simulink library "HIL_GenSet"  (Simulink 7.8)
settings: Solver=ode45  StartTime=0.0  StopTime=10.0  RelTol=1e-3
values from neighbouring files (symbols this model uses):
  Ts = 80e-6    (= 8e-05)    [global_parameters.m]    (also in scopeBuffer.m)
undefined symbols (not defined in the file or in its folder): DiscIntNeverNeededParam, Ts_Power
libraries: simulink x77, powerlib x55, discretizing x28
(part 2 of 9)

== system HIL_GenSet/GenSet_3p5MW_RTLAB_07082015/Generator with  Primary Controllers ==
  note: Mirjana M: Parameters for this generators are preset parameters from SimPower System for 72.5kVAr
  wref : Inport
  Vtref : Inport  Port=2
  Enable : Inport  Port=3
  w_meas_Woodward : Inport  Port=4
  V_meas_Woodward : Inport  Port=5
  72.5 kva Diesel Engine Speed & Voltage Control fast : Subsystem
  Scope2 : Scope  NumInputPorts=2
      settings: YMin=0.949571~0.99979  YMax=1.04953~1  SaveName=ScopeData6
  Synchronous Machine pu Fundamental : powerlib/Machines/Synchronous Machine pu Fundamental  PresetModel=No  MechanicalLoad=Mechanical power Pm  ShowDetailedParameters=on  RotorType=Salient-pole  NominalParameters=[4.375+006 460 60]  Stator=[0.008979 0.05 2.35 1.72]  Field=[0.00206 0.511]  Dampers2=[0.0652, 0.5134, 0.0287, 0.2553, 7.765e-3, 0.9167 ]  Dampers1=[0.2826 3.738 0.02545 0.2392]  Mechanical=[0.3468 0.009238 2]  PolePairs=2  InitialConditions="[ 0  0  0  0  0  0  0  0  0 ]"  SetSaturation=off  Saturation=[0.6404,0.7127,0.8441,0.9214,0.9956,1.082,1.19,1.316,1.457;0.7,0.7698,0.8872,0.9466,0.9969,1.046,1.1,1.151,1.201]  Units=per unit fundamental parameters  LoadFlowParameters=[1,0,0,0,0]  TsPowergui=0  TsBlock=-1  IterativeModel=Forward Euler  BusType=PV  Pref=0  Qref=0  Qmin=-inf  Qmax=inf  PLF=0  QLF=0
  A : PMIOPort  Port=1  Side=Right
  B : PMIOPort  Port=2  Side=Right
  C : PMIOPort  Port=3  Side=Right
  m : Outport
  wires:
  Enable/1 -> 72.5 kva Diesel Engine Speed & Voltage Control fast/3(Generator Enable)
  Vtref/1 -> 72.5 kva Diesel Engine Speed & Voltage Control fast/2(Vtref)
  wref/1 -> 72.5 kva Diesel Engine Speed & Voltage Control fast/1(wref)
  72.5 kva Diesel Engine Speed & Voltage Control fast/3(Vt) -> Scope2/1  "vt"
  72.5 kva Diesel Engine Speed & Voltage Control fast/4(w) -> Scope2/2  "w"
  Synchronous Machine pu Fundamental/1 -> m/1, 72.5 kva Diesel Engine Speed & Voltage Control fast/4(m)
  72.5 kva Diesel Engine Speed & Voltage Control fast/2(Vf) -> Synchronous Machine pu Fundamental/2
  72.5 kva Diesel Engine Speed & Voltage Control fast/1(Pm) -> Synchronous Machine pu Fundamental/1
  w_meas_Woodward/1 -> 72.5 kva Diesel Engine Speed & Voltage Control fast/5(w_meas_Wood)
  V_meas_Woodward/1 -> 72.5 kva Diesel Engine Speed & Voltage Control fast/6(V_meas_Wood)
  connections:
  C/RConn1 -- Synchronous Machine pu Fundamental/RConn3
  B/RConn1 -- Synchronous Machine pu Fundamental/RConn2
  A/RConn1 -- Synchronous Machine pu Fundamental/RConn1

== system HIL_GenSet/GenSet_3p5MW_RTLAB_07082015/Interface between Woodward Controller and simated generator ==
  note: Note: This may need a different scaling because it is the reference signal.
      | Reference has to be between 0.95 and 1.05 pu in order to be in tolerance.
  Woodward for wref : Inport
  Woodward for Vref : Inport  Port=2
  Add2 : Sum
  Add3 : Sum
  Gain2 : Gain  Gain=0.01
  Gain3 : Gain  Gain=0.01
  Mux1 : Mux  Inputs=2
  Vref_set : Constant
  wref_set : Constant
  wref,Vref : Outport
  wires:
  Gain2/1 -> Add2/1  "bias"
  Add2/1 -> Mux1/1
  wref_set/1 -> Add2/2
  Gain3/1 -> Add3/1  "bias"
  Vref_set/1 -> Add3/2
  Add3/1 -> Mux1/2
  Woodward for wref/1 -> Gain2/1
  Mux1/1 -> wref,Vref/1  "hardware"
  Woodward for Vref/1 -> Gain3/1

== system HIL_GenSet/GenSet_3p5MW_RTLAB_07082015/Simulated Generator Controller 3.5 MW ==
  Pref : Inport
  Qref : Inport  Port=2
  mode : Inport  Port=3
  set_vtref : Inport  Port=4
  set_wref : Inport  Port=5
  gen_m : Inport  Port=6
  Bus Selector1 : BusSelector  OutputSignals="Output active power   Peo (pu),Output reactive power  Qeo (pu)"
  Multiport Switch : MultiPortSwitch  zeroidx=off
  Mux1 : Mux  Inputs=2
  Mux2 : Mux  Inputs=2
  Mux3 : Mux  Inputs=2
  PQ control : Subsystem
  PV control : Subsystem
  "wref, Vref" : Outport
  wires:
  Bus Selector1/1 -> PQ control/2(P (pu)), PV control/2(P (pu))  "<Output active power   Peo (pu)>"
  gen_m/1 -> Bus Selector1/1
  PQ control/1(w_ref (pu)) -> Mux1/1
  PQ control/2(V_ref (pu)) -> Mux1/2
  PV control/1(w_ref (pu)) -> Mux2/1
  set_vtref/1 -> Mux2/2, Mux3/2
  Mux1/1 -> Multiport Switch/2
  Mux2/1 -> Multiport Switch/3
  Mux3/1 -> Multiport Switch/4
  Pref/1 -> PQ control/1(P_ref (pu)), PV control/1(P_ref (pu))
  Bus Selector1/2 -> PQ control/4(Q (pu))  "<Output reactive power  Qeo (pu)>"
  set_wref/1 -> Mux3/1
  Qref/1 -> PQ control/3(Q_ref (pu))
  mode/1 -> Multiport Switch/1
  Multiport Switch/1 -> "wref, Vref"/1

== system HIL_GenSet/GenSet_3p5MW_nPID_Manual_RTLAB/Generator with  Primary Controllers ==
  wref : Inport
  Vtref : Inport  Port=2
  Enable : Inport  Port=3
  72.5 kva Diesel Engine Speed & Voltage Control fast : Subsystem
  Scope2 : Scope  NumInputPorts=2
      settings: YMin=0~0.93  YMax=1.05~1.12  SaveName=ScopeData6
  Synchronous Machine pu Fundamental : powerlib/Machines/Synchronous Machine pu Fundamental  PresetModel=No  MechanicalLoad=Mechanical power Pm  ShowDetailedParameters=on  RotorType=Salient-pole  NominalParameters=[4e+006 460 60]  Stator=[0.008979 0.05 2.35 1.72]  Field=[0.00206 0.511]  Dampers2=[0.0652, 0.5134, 0.0287, 0.2553, 7.765e-3, 0.9167 ]  Dampers1=[0.2826 3.738 0.02545 0.2392]  Mechanical=[0.3468 0.009238 2]  PolePairs=2  InitialConditions="[ 0  0  0  0  0  0  0  0  0 ]"  SetSaturation=off  Saturation=[0.6404,0.7127,0.8441,0.9214,0.9956,1.082,1.19,1.316,1.457;0.7,0.7698,0.8872,0.9466,0.9969,1.046,1.1,1.151,1.201]  Units=per unit fundamental parameters  LoadFlowParameters=[1,0,0,0,0]  TsPowergui=0  TsBlock=-1  IterativeModel=Forward Euler  BusType=PV  Pref=0  Qref=0  Qmin=-inf  Qmax=inf  PLF=0  QLF=0
  A : PMIOPort  Port=1  Side=Right
  B : PMIOPort  Port=2  Side=Right
  C : PMIOPort  Port=3  Side=Right
  m : Outport
  wires:
  Enable/1 -> 72.5 kva Diesel Engine Speed & Voltage Control fast/3(Generator Enable)
  Vtref/1 -> 72.5 kva Diesel Engine Speed & Voltage Control fast/2(Vtref)
  wref/1 -> 72.5 kva Diesel Engine Speed & Voltage Control fast/1(wref)
  72.5 kva Diesel Engine Speed & Voltage Control fast/3(Vt) -> Scope2/1  "vt"
  72.5 kva Diesel Engine Speed & Voltage Control fast/4(w) -> Scope2/2  "w"
  Synchronous Machine pu Fundamental/1 -> m/1, 72.5 kva Diesel Engine Speed & Voltage Control fast/4(m)
  72.5 kva Diesel Engine Speed & Voltage Control fast/2(Vf) -> Synchronous Machine pu Fundamental/2
  72.5 kva Diesel Engine Speed & Voltage Control fast/1(Pm) -> Synchronous Machine pu Fundamental/1
  connections:
  C/RConn1 -- Synchronous Machine pu Fundamental/RConn3
  B/RConn1 -- Synchronous Machine pu Fundamental/RConn2
  A/RConn1 -- Synchronous Machine pu Fundamental/RConn1

== system HIL_GenSet/GenSet_3p5MW_nPID_Manual_RTLAB/Simulated Generator Controller 3.5 MW ==
  Pref : Inport
  Qref : Inport  Port=2
  mode : Inport  Port=3
  set_vtref : Inport  Port=4
  set_wref : Inport  Port=5
  gen_m : Inport  Port=6
  Bus Selector1 : BusSelector  OutputSignals="Output active power   Peo (pu),Output reactive power  Qeo (pu)"
  Multiport Switch : MultiPortSwitch  zeroidx=off
  Mux1 : Mux  Inputs=2
  Mux2 : Mux  Inputs=2
  Mux3 : Mux  Inputs=2
  PQ control : Subsystem
  PV control : Subsystem
  "wref, Vref" : Outport
  wires:
  Bus Selector1/1 -> PQ control/2(P (pu)), PV control/2(P (pu))  "<Output active power   Peo (pu)>"
  gen_m/1 -> Bus Selector1/1
  PQ control/1(w_ref (pu)) -> Mux1/1
  PQ control/2(V_ref (pu)) -> Mux1/2
  PV control/1(w_ref (pu)) -> Mux2/1
  set_vtref/1 -> Mux2/2, Mux3/2
  Mux1/1 -> Multiport Switch/2
  Mux2/1 -> Multiport Switch/3
  Mux3/1 -> Multiport Switch/4
  Pref/1 -> PQ control/1(P_ref (pu)), PV control/1(P_ref (pu))
  Bus Selector1/2 -> PQ control/4(Q (pu))  "<Output reactive power  Qeo (pu)>"
  set_wref/1 -> Mux3/1
  Qref/1 -> PQ control/3(Q_ref (pu))
  mode/1 -> Multiport Switch/1
  Multiport Switch/1 -> "wref, Vref"/1

== system HIL_GenSet/GenSet_3p5MW_new_PID_RTLAB/60kW Generator with  Primary Controllers ==
  note: Mirjana M: Parameters for this generators are preset parameters from SimPower System for 72.5kVAr
  wref : Inport
  Vtref : Inport  Port=2
  Enable : Inport  Port=3
  w_meas_Woodward : Inport  Port=4
  V_meas_Woodward : Inport  Port=5
  72.5 kva Diesel Engine Speed & Voltage Control fast : Subsystem
  Scope2 : Scope  NumInputPorts=2
      settings: YMin=0.949571~0.99979  YMax=1.04953~1  SaveName=ScopeData6
  Synchronous Machine pu Fundamental : powerlib/Machines/Synchronous Machine pu Fundamental  PresetModel=No  MechanicalLoad=Mechanical power Pm  ShowDetailedParameters=on  RotorType=Salient-pole  NominalParameters=[4.375+006 460 60]  Stator=[0.008979 0.05 2.35 1.72]  Field=[0.00206 0.511]  Dampers2=[0.0652, 0.5134, 0.0287, 0.2553, 7.765e-3, 0.9167 ]  Dampers1=[0.2826 3.738 0.02545 0.2392]  Mechanical=[0.3468 0.009238 2]  PolePairs=2  InitialConditions="[ 0  0  0  0  0  0  0  0  0 ]"  SetSaturation=off  Saturation=[0.6404,0.7127,0.8441,0.9214,0.9956,1.082,1.19,1.316,1.457;0.7,0.7698,0.8872,0.9466,0.9969,1.046,1.1,1.151,1.201]  Units=per unit fundamental parameters  LoadFlowParameters=[1,0,0,0,0]  TsPowergui=0  TsBlock=-1  IterativeModel=Forward Euler  BusType=PV  Pref=0  Qref=0  Qmin=-inf  Qmax=inf  PLF=0  QLF=0
  A : PMIOPort  Port=1  Side=Right
  B : PMIOPort  Port=2  Side=Right
  C : PMIOPort  Port=3  Side=Right
  m : Outport
  wires:
  Enable/1 -> 72.5 kva Diesel Engine Speed & Voltage Control fast/3(Generator Enable)
  Vtref/1 -> 72.5 kva Diesel Engine Speed & Voltage Control fast/2(Vtref)
  wref/1 -> 72.5 kva Diesel Engine Speed & Voltage Control fast/1(wref)
  72.5 kva Diesel Engine Speed & Voltage Control fast/3(Vt) -> Scope2/1
  72.5 kva Diesel Engine Speed & Voltage Control fast/4(w) -> Scope2/2
  Synchronous Machine pu Fundamental/1 -> m/1, 72.5 kva Diesel Engine Speed & Voltage Control fast/4(m)
  72.5 kva Diesel Engine Speed & Voltage Control fast/2(Vf) -> Synchronous Machine pu Fundamental/2
  72.5 kva Diesel Engine Speed & Voltage Control fast/1(Pm) -> Synchronous Machine pu Fundamental/1
  w_meas_Woodward/1 -> 72.5 kva Diesel Engine Speed & Voltage Control fast/5(w_meas_Wood)
  V_meas_Woodward/1 -> 72.5 kva Diesel Engine Speed & Voltage Control fast/6(V_meas_Wood)
  connections:
  C/RConn1 -- Synchronous Machine pu Fundamental/RConn3
  B/RConn1 -- Synchronous Machine pu Fundamental/RConn2
  A/RConn1 -- Synchronous Machine pu Fundamental/RConn1

== system HIL_GenSet/GenSet_3p5MW_new_PID_RTLAB/Interface between Woodward Controller and simated generator ==
  note: Note: This may need a different scaling because it is the reference signal.
      | Reference has to be between 0.95 and 1.05 pu in order to be in tolerance.
  Woodward for wref : Inport
  Woodward for Vref : Inport  Port=2
  Add2 : Sum
  Add3 : Sum
  Gain2 : Gain  Gain=0.005
  Gain3 : Gain  Gain=0.005
  Mux1 : Mux  Inputs=2
  Vref_set : Constant
  wref_set : Constant
  wref,Vref : Outport
  wires:
  Gain2/1 -> Add2/1  "bias"
  Add2/1 -> Mux1/1
  wref_set/1 -> Add2/2
  Gain3/1 -> Add3/1  "bias"
  Vref_set/1 -> Add3/2
  Add3/1 -> Mux1/2
  Woodward for wref/1 -> Gain2/1
  Mux1/1 -> wref,Vref/1  "hardware"
  Woodward for Vref/1 -> Gain3/1

== system HIL_GenSet/GenSet_3p5MW_new_PID_RTLAB/Simulated Generator Controller ==
  Bus Selector1 : BusSelector  OutputSignals="Output active power   Peo (pu),Output reactive power  Qeo (pu)"
  Multiport Switch : MultiPortSwitch  zeroidx=off
  Mux1 : Mux  Inputs=2
  Mux2 : Mux  Inputs=2
  Mux3 : Mux  Inputs=2
  PQ control : Subsystem
  PV control : Subsystem
  Pref : Constant  Value=set_Pref
  Qref : Constant  Value=set_Qref
  mode (1-3) : Constant  Value=mode
  set_vtref : Constant  Value=set_vref
  set_wref : Constant  Value=set_wref
  "wref, Vref" : Outport
  wires:
  Bus Selector1/1 -> PQ control/2(P (pu)), PV control/2(P (pu))  "<Output active power   Peo (pu)>"
  [gen_m] -> Bus Selector1/1
  PQ control/1(w_ref (pu)) -> Mux1/1
  PQ control/2(V_ref (pu)) -> Mux1/2
  PV control/1(w_ref (pu)) -> Mux2/1
  set_vtref/1 -> Mux2/2, Mux3/2
  Mux1/1 -> Multiport Switch/2
  Mux2/1 -> Multiport Switch/3
  Mux3/1 -> Multiport Switch/4
  Pref/1 -> PQ control/1(P_ref (pu)), PV control/1(P_ref (pu))
  Bus Selector1/2 -> PQ control/4(Q (pu))  "<Output reactive power  Qeo (pu)>"
  set_wref/1 -> Mux3/1
  Qref/1 -> PQ control/3(Q_ref (pu))
  mode (1-3)/1 -> Multiport Switch/1
  Multiport Switch/1 -> "wref, Vref"/1

== system HIL_GenSet/GenSet_4MW_14kV/Generator with  Primary Controllers ==
  wref : Inport
  Vtref : Inport  Port=2
  Enable : Inport  Port=3
  72.5 kva Diesel Engine Speed & Voltage Control fast : Subsystem
  Synchronous Machine pu Fundamental : powerlib/Machines/Synchronous Machine pu Fundamental  PresetModel=No  MechanicalLoad=Mechanical power Pm  ShowDetailedParameters=on  RotorType=Salient-pole  NominalParameters=[4e+006 13800 60]  Stator=[0.008979 0.05 2.35 1.72]  Field=[0.00206 0.511]  Dampers2=[0.0652, 0.5134, 0.0287, 0.2553, 7.765e-3, 0.9167 ]  Dampers1=[0.2826 3.738 0.02545 0.2392]  Mechanical=[0.3468 0.009238 2]  PolePairs=2  InitialConditions="[ 0  0  0  0  0  0  0  0  0 ]"  SetSaturation=off  Saturation=[0.6404,0.7127,0.8441,0.9214,0.9956,1.082,1.19,1.316,1.457;0.7,0.7698,0.8872,0.9466,0.9969,1.046,1.1,1.151,1.201]  Units=per unit fundamental parameters  LoadFlowParameters=[1,0,0,0,0]  TsPowergui=0  TsBlock=-1  IterativeModel=Forward Euler  BusType=PV  Pref=0  Qref=0  Qmin=-inf  Qmax=inf  PLF=0  QLF=0
  Terminator : Terminator
  Terminator1 : Terminator
  A : PMIOPort  Port=1  Side=Right
  B : PMIOPort  Port=2  Side=Right
  C : PMIOPort  Port=3  Side=Right
  m : Outport
  wires:
  Enable/1 -> 72.5 kva Diesel Engine Speed & Voltage Control fast/3(Generator Enable)
  Vtref/1 -> 72.5 kva Diesel Engine Speed & Voltage Control fast/2(Vtref)
  wref/1 -> 72.5 kva Diesel Engine Speed & Voltage Control fast/1(wref)
  Synchronous Machine pu Fundamental/1 -> m/1, 72.5 kva Diesel Engine Speed & Voltage Control fast/4(m)
  72.5 kva Diesel Engine Speed & Voltage Control fast/2(Vf) -> Synchronous Machine pu Fundamental/2
  72.5 kva Diesel Engine Speed & Voltage Control fast/1(Pm) -> Synchronous Machine pu Fundamental/1
  72.5 kva Diesel Engine Speed & Voltage Control fast/3(Vt) -> Terminator/1  "vt"
  72.5 kva Diesel Engine Speed & Voltage Control fast/4(w) -> Terminator1/1  "w"
  connections:
  C/RConn1 -- Synchronous Machine pu Fundamental/RConn3
  B/RConn1 -- Synchronous Machine pu Fundamental/RConn2
  A/RConn1 -- Synchronous Machine pu Fundamental/RConn1

== system HIL_GenSet/GenSet_4MW_14kV/NumOscillation ==
  Ground2 : powerlib/Elements/Ground  LConnTagsString=a
  "RLC " : powerlib/Elements/Parallel RLC Branch  LConnTagsString=a  RConnTagsString=__new0  BranchType=R  Resistance=10e6  Inductance=inf  SetiL0=off  InitialCurrent=0  Capacitance=10e-6  Setx0=off  InitialVoltage=0  Measurements=None
  RLC1 : powerlib/Elements/Parallel RLC Branch  LConnTagsString=a  RConnTagsString=__new0  BranchType=R  Resistance=10e6  Inductance=inf  SetiL0=off  InitialCurrent=0  Capacitance=10e-6  Setx0=off  InitialVoltage=0  Measurements=None
  RLC2 : powerlib/Elements/Parallel RLC Branch  LConnTagsString=a  RConnTagsString=__new0  BranchType=R  Resistance=10e6  Inductance=inf  SetiL0=off  InitialCurrent=0  Capacitance=10e-6  Setx0=off  InitialVoltage=0  Measurements=None
  RLC3 : powerlib/Elements/Parallel RLC Branch  LConnTagsString=a  RConnTagsString=__new0  BranchType=R  Resistance=10e-3  Inductance=inf  SetiL0=off  InitialCurrent=0  Capacitance=0  Setx0=off  InitialVoltage=0  Measurements=None
  RLC4 : powerlib/Elements/Parallel RLC Branch  LConnTagsString=a  RConnTagsString=__new0  BranchType=R  Resistance=10e-3  Inductance=inf  SetiL0=off  InitialCurrent=0  Capacitance=0  Setx0=off  InitialVoltage=0  Measurements=None
  RLC5 : powerlib/Elements/Parallel RLC Branch  LConnTagsString=a  RConnTagsString=__new0  BranchType=R  Resistance=10e-3  Inductance=inf  SetiL0=off  InitialCurrent=0  Capacitance=0  Setx0=off  InitialVoltage=0  Measurements=None
  A : PMIOPort  Port=1  Side=Left
  B : PMIOPort  Port=2  Side=Left
  C : PMIOPort  Port=3  Side=Left
  connections:
  C/RConn1 -- RLC5/LConn1
  B/RConn1 -- RLC4/LConn1
  A/RConn1 -- RLC3/LConn1
  RLC3/RConn1 -- RLC2/LConn1
  RLC1/LConn1 -- RLC4/RConn1
  "RLC "/LConn1 -- RLC5/RConn1
  RLC2/RConn1 -- Ground2/LConn1 -- RLC1/RConn1 -- "RLC "/RConn1

== system HIL_GenSet/GenSet_4MW_14kV/Simulated Generator Controller 3.5 MW ==
  Pref : Inport
  Qref : Inport  Port=2
  mode : Inport  Port=3
  set_vtref : Inport  Port=4
  set_wref : Inport  Port=5
  gen_m : Inport  Port=6
  Bus Selector1 : BusSelector  OutputSignals="Output active power   Peo (pu),Output reactive power  Qeo (pu)"
  Multiport Switch : MultiPortSwitch  zeroidx=off
  Mux1 : Mux  Inputs=2
  Mux2 : Mux  Inputs=2
  Mux3 : Mux  Inputs=2
  PQ control : Subsystem
  PV control : Subsystem
  "wref, Vref" : Outport
  wires:
  Bus Selector1/1 -> PQ control/2(P (pu)), PV control/2(P (pu))  "<Output active power   Peo (pu)>"
  gen_m/1 -> Bus Selector1/1
  PQ control/1(w_ref (pu)) -> Mux1/1
  PQ control/2(V_ref (pu)) -> Mux1/2
  PV control/1(w_ref (pu)) -> Mux2/1
  set_vtref/1 -> Mux2/2, Mux3/2
  Mux1/1 -> Multiport Switch/2
  Mux2/1 -> Multiport Switch/3
  Mux3/1 -> Multiport Switch/4
  Pref/1 -> PQ control/1(P_ref (pu)), PV control/1(P_ref (pu))
  Bus Selector1/2 -> PQ control/4(Q (pu))  "<Output reactive power  Qeo (pu)>"
  set_wref/1 -> Mux3/1
  Qref/1 -> PQ control/3(Q_ref (pu))
  mode/1 -> Multiport Switch/1
  Multiport Switch/1 -> "wref, Vref"/1

== system HIL_GenSet/GenSet_4MW_14kV_07232015/Generator with  Primary Controllers ==
  wref : Inport
  Vtref : Inport  Port=2
  Enable : Inport  Port=3
  Diesel Engine Speed & Voltage Control fast : Subsystem
  Synchronous Machine pu Fundamental : powerlib/Machines/Synchronous Machine pu Fundamental  PresetModel=No  MechanicalLoad=Mechanical power Pm  ShowDetailedParameters=on  RotorType=Salient-pole  NominalParameters=[4e+006 13800 60]  Stator=[0.008979 0.05 2.35 1.72]  Field=[0.00206 0.511]  Dampers2=[0.0652, 0.5134, 0.0287, 0.2553, 7.765e-3, 0.9167 ]  Dampers1=[0.2826 3.738 0.02545 0.2392]  Mechanical=[0.3468 0.009238 2]  PolePairs=2  InitialConditions="[ 0  0  0  0  0  0  0  0  0 ]"  SetSaturation=off  Saturation=[0.6404,0.7127,0.8441,0.9214,0.9956,1.082,1.19,1.316,1.457;0.7,0.7698,0.8872,0.9466,0.9969,1.046,1.1,1.151,1.201]  Units=per unit fundamental parameters  LoadFlowParameters=[1,0,0,0,0]  TsPowergui=0  TsBlock=-1  IterativeModel=Forward Euler  BusType=PV  Pref=0  Qref=0  Qmin=-inf  Qmax=inf  PLF=0  QLF=0
  Terminator : Terminator
  Terminator1 : Terminator
  A : PMIOPort  Port=1  Side=Right
  B : PMIOPort  Port=2  Side=Right
  C : PMIOPort  Port=3  Side=Right
  m : Outport
  wires:
  Enable/1 -> Diesel Engine Speed & Voltage Control fast/3(Generator Enable)
  Vtref/1 -> Diesel Engine Speed & Voltage Control fast/2(Vtref)
  wref/1 -> Diesel Engine Speed & Voltage Control fast/1(wref)
  Synchronous Machine pu Fundamental/1 -> m/1, Diesel Engine Speed & Voltage Control fast/4(m)
  Diesel Engine Speed & Voltage Control fast/2(Vf) -> Synchronous Machine pu Fundamental/2
  Diesel Engine Speed & Voltage Control fast/1(Pm) -> Synchronous Machine pu Fundamental/1
  Diesel Engine Speed & Voltage Control fast/3(Vt) -> Terminator/1  "vt"
  Diesel Engine Speed & Voltage Control fast/4(w) -> Terminator1/1  "w"
  connections:
  C/RConn1 -- Synchronous Machine pu Fundamental/RConn3
  B/RConn1 -- Synchronous Machine pu Fundamental/RConn2
  A/RConn1 -- Synchronous Machine pu Fundamental/RConn1

== system HIL_GenSet/GenSet_4MW_14kV_07232015/NumOscillation ==
  Ground2 : powerlib/Elements/Ground  LConnTagsString=a
  "RLC " : powerlib/Elements/Parallel RLC Branch  LConnTagsString=a  RConnTagsString=__new0  BranchType=R  Resistance=10e6  Inductance=inf  SetiL0=off  InitialCurrent=0  Capacitance=10e-6  Setx0=off  InitialVoltage=0  Measurements=None
  RLC1 : powerlib/Elements/Parallel RLC Branch  LConnTagsString=a  RConnTagsString=__new0  BranchType=R  Resistance=10e6  Inductance=inf  SetiL0=off  InitialCurrent=0  Capacitance=10e-6  Setx0=off  InitialVoltage=0  Measurements=None
  RLC2 : powerlib/Elements/Parallel RLC Branch  LConnTagsString=a  RConnTagsString=__new0  BranchType=R  Resistance=10e6  Inductance=inf  SetiL0=off  InitialCurrent=0  Capacitance=10e-6  Setx0=off  InitialVoltage=0  Measurements=None
  RLC3 : powerlib/Elements/Parallel RLC Branch  LConnTagsString=a  RConnTagsString=__new0  BranchType=R  Resistance=10e-3  Inductance=inf  SetiL0=off  InitialCurrent=0  Capacitance=0  Setx0=off  InitialVoltage=0  Measurements=None
  RLC4 : powerlib/Elements/Parallel RLC Branch  LConnTagsString=a  RConnTagsString=__new0  BranchType=R  Resistance=10e-3  Inductance=inf  SetiL0=off  InitialCurrent=0  Capacitance=0  Setx0=off  InitialVoltage=0  Measurements=None
  RLC5 : powerlib/Elements/Parallel RLC Branch  LConnTagsString=a  RConnTagsString=__new0  BranchType=R  Resistance=10e-3  Inductance=inf  SetiL0=off  InitialCurrent=0  Capacitance=0  Setx0=off  InitialVoltage=0  Measurements=None
  A : PMIOPort  Port=1  Side=Left
  B : PMIOPort  Port=2  Side=Left
  C : PMIOPort  Port=3  Side=Left
  connections:
  C/RConn1 -- RLC5/LConn1
  B/RConn1 -- RLC4/LConn1
  A/RConn1 -- RLC3/LConn1
  RLC3/RConn1 -- RLC2/LConn1
  RLC1/LConn1 -- RLC4/RConn1
  "RLC "/LConn1 -- RLC5/RConn1
  RLC2/RConn1 -- Ground2/LConn1 -- RLC1/RConn1 -- "RLC "/RConn1

== system HIL_GenSet/GenSet_4MW_14kV_07232015/Simulated Generator Controller 3.5 MW ==
  Pref : Inport
  Qref : Inport  Port=2
  mode : Inport  Port=3
  set_vtref : Inport  Port=4
  set_wref : Inport  Port=5
  gen_m : Inport  Port=6
  Bus Selector1 : BusSelector  OutputSignals="Output active power   Peo (pu),Output reactive power  Qeo (pu)"
  Multiport Switch : MultiPortSwitch  zeroidx=off
  Mux1 : Mux  Inputs=2
  Mux2 : Mux  Inputs=2
  Mux3 : Mux  Inputs=2
  PQ control : Subsystem
  PV control : Subsystem
  "wref, Vref" : Outport
  wires:
  Bus Selector1/1 -> PQ control/2(P (pu)), PV control/2(P (pu))  "<Output active power   Peo (pu)>"
  gen_m/1 -> Bus Selector1/1
  PQ control/1(w_ref (pu)) -> Mux1/1
  PQ control/2(V_ref (pu)) -> Mux1/2
  PV control/1(w_ref (pu)) -> Mux2/1
  set_vtref/1 -> Mux2/2, Mux3/2
  Mux1/1 -> Multiport Switch/2
  Mux2/1 -> Multiport Switch/3
  Mux3/1 -> Multiport Switch/4
  Pref/1 -> PQ control/1(P_ref (pu)), PV control/1(P_ref (pu))
  Bus Selector1/2 -> PQ control/4(Q (pu))  "<Output reactive power  Qeo (pu)>"
  set_wref/1 -> Mux3/1
  Qref/1 -> PQ control/3(Q_ref (pu))
  mode/1 -> Multiport Switch/1
  Multiport Switch/1 -> "wref, Vref"/1

== system HIL_GenSet/GenSet_4MW_14kV_07232015/StabilityL ==
  Constant Load : powerlib/Elements/Three-Phase Parallel RLC Load  LConnTagsString=A|B|C  Configuration=Y (grounded)  NominalVoltage=v  NominalFrequency=60  ActivePower=kVA*1E3*pf  InductivePower=kVA*1E3*sqrt(1-pf^2)  CapacitivePower=0  Measurements=None  LoadType=constant Z
  A : PMIOPort  Port=1  Side=Left
  B : PMIOPort  Port=2  Side=Left
  C : PMIOPort  Port=3  Side=Left
  connections:
  A/RConn1 -- Constant Load/LConn1
  B/RConn1 -- Constant Load/LConn2
  C/RConn1 -- Constant Load/LConn3

== system HIL_GenSet/GenSet_4MW_14kV_09022015/Generator with  Primary Controllers ==
  wref : Inport
  Vtref : Inport  Port=2
  Enable : Inport  Port=3
  Diesel Engine Speed & Voltage Control fast : Subsystem
  Synchronous Machine pu Fundamental : powerlib/Machines/Synchronous Machine pu Fundamental  PresetModel=No  MechanicalLoad=Mechanical power Pm  ShowDetailedParameters=on  RotorType=Salient-pole  NominalParameters=[4e+006 13800 60]  Stator=[0.008979 0.05 2.35 1.72]  Field=[0.00206 0.511]  Dampers2=[0.0652, 0.5134, 0.0287, 0.2553, 7.765e-3, 0.9167 ]  Dampers1=[0.2826 3.738 0.02545 0.2392]  Mechanical=[0.3468 0.009238 2]  PolePairs=2  InitialConditions="[ 0  0  0  0  0  0  0  0  0 ]"  SetSaturation=off  Saturation=[0.6404,0.7127,0.8441,0.9214,0.9956,1.082,1.19,1.316,1.457;0.7,0.7698,0.8872,0.9466,0.9969,1.046,1.1,1.151,1.201]  Units=per unit fundamental parameters  LoadFlowParameters=[1,0,0,0,0]  TsPowergui=0  TsBlock=-1  IterativeModel=Forward Euler  BusType=PV  Pref=0  Qref=0  Qmin=-inf  Qmax=inf  PLF=0  QLF=0
  Terminator : Terminator
  Terminator1 : Terminator
  A : PMIOPort  Port=1  Side=Right
  B : PMIOPort  Port=2  Side=Right
  C : PMIOPort  Port=3  Side=Right
  m : Outport
  wires:
  Enable/1 -> Diesel Engine Speed & Voltage Control fast/3(Generator Enable)
  Vtref/1 -> Diesel Engine Speed & Voltage Control fast/2(Vtref)
  wref/1 -> Diesel Engine Speed & Voltage Control fast/1(wref)
  Synchronous Machine pu Fundamental/1 -> m/1, Diesel Engine Speed & Voltage Control fast/4(m)
  Diesel Engine Speed & Voltage Control fast/2(Vf) -> Synchronous Machine pu Fundamental/2
  Diesel Engine Speed & Voltage Control fast/1(Pm) -> Synchronous Machine pu Fundamental/1
  Diesel Engine Speed & Voltage Control fast/3(Vt) -> Terminator/1  "vt"
  Diesel Engine Speed & Voltage Control fast/4(w) -> Terminator1/1  "w"
  connections:
  C/RConn1 -- Synchronous Machine pu Fundamental/RConn3
  B/RConn1 -- Synchronous Machine pu Fundamental/RConn2
  A/RConn1 -- Synchronous Machine pu Fundamental/RConn1

== system HIL_GenSet/GenSet_4MW_14kV_09022015/NumOscillation ==
  Ground2 : powerlib/Elements/Ground  LConnTagsString=a
  "RLC " : powerlib/Elements/Parallel RLC Branch  LConnTagsString=a  RConnTagsString=__new0  BranchType=R  Resistance=10e6  Inductance=inf  SetiL0=off  InitialCurrent=0  Capacitance=10e-6  Setx0=off  InitialVoltage=0  Measurements=None
  RLC1 : powerlib/Elements/Parallel RLC Branch  LConnTagsString=a  RConnTagsString=__new0  BranchType=R  Resistance=10e6  Inductance=inf  SetiL0=off  InitialCurrent=0  Capacitance=10e-6  Setx0=off  InitialVoltage=0  Measurements=None
  RLC2 : powerlib/Elements/Parallel RLC Branch  LConnTagsString=a  RConnTagsString=__new0  BranchType=R  Resistance=10e6  Inductance=inf  SetiL0=off  InitialCurrent=0  Capacitance=10e-6  Setx0=off  InitialVoltage=0  Measurements=None
  RLC3 : powerlib/Elements/Parallel RLC Branch  LConnTagsString=a  RConnTagsString=__new0  BranchType=R  Resistance=10e-3  Inductance=inf  SetiL0=off  InitialCurrent=0  Capacitance=0  Setx0=off  InitialVoltage=0  Measurements=None
  RLC4 : powerlib/Elements/Parallel RLC Branch  LConnTagsString=a  RConnTagsString=__new0  BranchType=R  Resistance=10e-3  Inductance=inf  SetiL0=off  InitialCurrent=0  Capacitance=0  Setx0=off  InitialVoltage=0  Measurements=None
  RLC5 : powerlib/Elements/Parallel RLC Branch  LConnTagsString=a  RConnTagsString=__new0  BranchType=R  Resistance=10e-3  Inductance=inf  SetiL0=off  InitialCurrent=0  Capacitance=0  Setx0=off  InitialVoltage=0  Measurements=None
  A : PMIOPort  Port=1  Side=Left
  B : PMIOPort  Port=2  Side=Left
  C : PMIOPort  Port=3  Side=Left
  connections:
  C/RConn1 -- RLC5/LConn1
  B/RConn1 -- RLC4/LConn1
  A/RConn1 -- RLC3/LConn1
  RLC3/RConn1 -- RLC2/LConn1
  RLC1/LConn1 -- RLC4/RConn1
  "RLC "/LConn1 -- RLC5/RConn1
  RLC2/RConn1 -- Ground2/LConn1 -- RLC1/RConn1 -- "RLC "/RConn1

== system HIL_GenSet/GenSet_4MW_14kV_09022015/Simulated Generator Controller 3.5 MW ==
  Pref : Inport
  Qref : Inport  Port=2
  mode : Inport  Port=3
  set_vtref : Inport  Port=4
  set_wref : Inport  Port=5
  gen_m : Inport  Port=6
  Bus Selector1 : BusSelector  OutputSignals="Output active power   Peo (pu),Output reactive power  Qeo (pu)"
  Multiport Switch : MultiPortSwitch  zeroidx=off
  Mux1 : Mux  Inputs=2
  Mux2 : Mux  Inputs=2
  Mux3 : Mux  Inputs=2
  PQ control : Subsystem
  PV control : Subsystem
  "wref, Vref" : Outport
  wires:
  Bus Selector1/1 -> PQ control/2(P (pu)), PV control/2(P (pu))  "<Output active power   Peo (pu)>"
  gen_m/1 -> Bus Selector1/1
  PQ control/1(w_ref (pu)) -> Mux1/1
  PQ control/2(V_ref (pu)) -> Mux1/2
  PV control/1(w_ref (pu)) -> Mux2/1
  set_vtref/1 -> Mux2/2, Mux3/2
  Mux1/1 -> Multiport Switch/2
  Mux2/1 -> Multiport Switch/3
  Mux3/1 -> Multiport Switch/4
  Pref/1 -> PQ control/1(P_ref (pu)), PV control/1(P_ref (pu))
  Bus Selector1/2 -> PQ control/4(Q (pu))  "<Output reactive power  Qeo (pu)>"
  set_wref/1 -> Mux3/1
  Qref/1 -> PQ control/3(Q_ref (pu))
  mode/1 -> Multiport Switch/1
  Multiport Switch/1 -> "wref, Vref"/1

== system HIL_GenSet/GenSet_4MW_14kV_09022015/StabilityL ==
  Constant Load : powerlib/Elements/Three-Phase Parallel RLC Load  LConnTagsString=A|B|C  Configuration=Y (grounded)  NominalVoltage=v  NominalFrequency=60  ActivePower=kVA*1E3*pf  InductivePower=kVA*1E3*sqrt(1-pf^2)  CapacitivePower=0  Measurements=None  LoadType=constant Z
  A : PMIOPort  Port=1  Side=Left
  B : PMIOPort  Port=2  Side=Left
  C : PMIOPort  Port=3  Side=Left
  connections:
  A/RConn1 -- Constant Load/LConn1
  B/RConn1 -- Constant Load/LConn2
  C/RConn1 -- Constant Load/LConn3

== system HIL_GenSet/GenSet_900kW_07232015/900kW Generator with  Primary Controllers ==
  note: Mirjana M: Parameters for this generators are preset parameters from SimPower System for 72.5kVAr
  wref : Inport
  Vtref : Inport  Port=2
  Enable : Inport  Port=3
  w_meas_Woodward : Inport  Port=4
  V_meas_Woodward : Inport  Port=5
  Diesel Engine Speed & Voltage Control fast : Subsystem
  Synchronous Machine pu Fundamental : powerlib/Machines/Synchronous Machine pu Fundamental  PresetModel=22: 60Hz 460V 1075kVA 1800RPM  MechanicalLoad=Mechanical power Pm  ShowDetailedParameters=on  RotorType=Salient-pole  NominalParameters=[1.075e+006 460 60]  Stator=[0.01524 0.08 2.81 1.64]  Field=[0.004319 0.531]  Dampers2=[0.0652, 0.5134, 0.0287, 0.2553, 7.765e-3, 0.9167 ]  Dampers1=[0.2343 2.655 0.03365 0.2408]  Mechanical=[0.3222 0.01322 2]  PolePairs=2  InitialConditions="[ 0  0  0  0  0  0  0  0  0 ]"  SetSaturation=off  Saturation=[0.6404,0.7127,0.8441,0.9214,0.9956,1.082,1.19,1.316,1.457;0.7,0.7698,0.8872,0.9466,0.9969,1.046,1.1,1.151,1.201]  Units=per unit fundamental parameters  LoadFlowParameters=[1,0,0,0,0]  TsPowergui=0  TsBlock=-1  IterativeModel=Forward Euler  BusType=PV  Pref=0  Qref=0  Qmin=-inf  Qmax=inf  PLF=0  QLF=0
  Terminator : Terminator
  Terminator1 : Terminator
  A : PMIOPort  Port=1  Side=Right
  B : PMIOPort  Port=2  Side=Right
  C : PMIOPort  Port=3  Side=Right
  m : Outport
  wires:
  Diesel Engine Speed & Voltage Control fast/4(w) -> Terminator1/1  "w"
  Diesel Engine Speed & Voltage Control fast/3(Vt) -> Terminator/1  "vt"
  Vtref/1 -> Diesel Engine Speed & Voltage Control fast/2(Vtref)
  wref/1 -> Diesel Engine Speed & Voltage Control fast/1(wref)
  Diesel Engine Speed & Voltage Control fast/2(Vf) -> Synchronous Machine pu Fundamental/2  "vf"
  Diesel Engine Speed & Voltage Control fast/1(Pm) -> Synchronous Machine pu Fundamental/1  "pm"
  Enable/1 -> Diesel Engine Speed & Voltage Control fast/3(Generator Enable)
  Synchronous Machine pu Fundamental/1 -> m/1, Diesel Engine Speed & Voltage Control fast/4(m)
  w_meas_Woodward/1 -> Diesel Engine Speed & Voltage Control fast/5(w_meas_Wood)
  V_meas_Woodward/1 -> Diesel Engine Speed & Voltage Control fast/6(V_meas_Wood)
  connections:
  C/RConn1 -- Synchronous Machine pu Fundamental/RConn3
  B/RConn1 -- Synchronous Machine pu Fundamental/RConn2
  A/RConn1 -- Synchronous Machine pu Fundamental/RConn1

== system HIL_GenSet/GenSet_900kW_07232015/Interface between Woodward Controller and simated generator ==
  note: Note: This may need a different scaling because it is the reference signal.
      | Reference has to be between 0.95 and 1.05 pu in order to be in tolerance.
  Woodward for wref : Inport
  Woodward for Vref : Inport  Port=2
  Add2 : Sum
  Add3 : Sum
  Gain2 : Gain  Gain=0.005
  Gain3 : Gain  Gain=0.005
  Mux1 : Mux  Inputs=2
  Vref_set : Constant
  wref_set : Constant
  wref,Vref : Outport
  wires:
  Gain2/1 -> Add2/1  "bias"
  Add2/1 -> Mux1/1
  wref_set/1 -> Add2/2
  Gain3/1 -> Add3/1  "bias"
  Vref_set/1 -> Add3/2
  Add3/1 -> Mux1/2
  Woodward for wref/1 -> Gain2/1
  Mux1/1 -> wref,Vref/1  "hardware"
  Woodward for Vref/1 -> Gain3/1

== system HIL_GenSet/GenSet_900kW_07232015/NumOscillation ==
  Ground2 : powerlib/Elements/Ground  LConnTagsString=a
  "RLC " : powerlib/Elements/Parallel RLC Branch  LConnTagsString=a  RConnTagsString=__new0  BranchType=R  Resistance=10e6  Inductance=inf  SetiL0=off  InitialCurrent=0  Capacitance=10e-6  Setx0=off  InitialVoltage=0  Measurements=None
  RLC1 : powerlib/Elements/Parallel RLC Branch  LConnTagsString=a  RConnTagsString=__new0  BranchType=R  Resistance=10e6  Inductance=inf  SetiL0=off  InitialCurrent=0  Capacitance=10e-6  Setx0=off  InitialVoltage=0  Measurements=None
  RLC2 : powerlib/Elements/Parallel RLC Branch  LConnTagsString=a  RConnTagsString=__new0  BranchType=R  Resistance=10e6  Inductance=inf  SetiL0=off  InitialCurrent=0  Capacitance=10e-6  Setx0=off  InitialVoltage=0  Measurements=None
  RLC3 : powerlib/Elements/Parallel RLC Branch  LConnTagsString=a  RConnTagsString=__new0  BranchType=R  Resistance=10e-3  Inductance=inf  SetiL0=off  InitialCurrent=0  Capacitance=0  Setx0=off  InitialVoltage=0  Measurements=None
  RLC4 : powerlib/Elements/Parallel RLC Branch  LConnTagsString=a  RConnTagsString=__new0  BranchType=R  Resistance=10e-3  Inductance=inf  SetiL0=off  InitialCurrent=0  Capacitance=0  Setx0=off  InitialVoltage=0  Measurements=None
  RLC5 : powerlib/Elements/Parallel RLC Branch  LConnTagsString=a  RConnTagsString=__new0  BranchType=R  Resistance=10e-3  Inductance=inf  SetiL0=off  InitialCurrent=0  Capacitance=0  Setx0=off  InitialVoltage=0  Measurements=None
  A : PMIOPort  Port=1  Side=Left
  B : PMIOPort  Port=2  Side=Left
  C : PMIOPort  Port=3  Side=Left
  connections:
  C/RConn1 -- RLC5/LConn1
  B/RConn1 -- RLC4/LConn1
  A/RConn1 -- RLC3/LConn1
  RLC3/RConn1 -- RLC2/LConn1
  RLC1/LConn1 -- RLC4/RConn1
  "RLC "/LConn1 -- RLC5/RConn1
  RLC2/RConn1 -- Ground2/LConn1 -- RLC1/RConn1 -- "RLC "/RConn1

== system HIL_GenSet/GenSet_900kW_07232015/Simulated Generator Controller 900 kW ==
  Pref : Inport
  Qref : Inport  Port=2
  mode : Inport  Port=3
  set_vtref : Inport  Port=4
  set_wref : Inport  Port=5
  gen_m : Inport  Port=6
  Bus Selector1 : BusSelector  OutputSignals="Output active power   Peo (pu),Output reactive power  Qeo (pu)"
  Multiport Switch : MultiPortSwitch  zeroidx=off
  Mux1 : Mux  Inputs=2
  Mux2 : Mux  Inputs=2
  Mux3 : Mux  Inputs=2
  PQ control : Subsystem
  PV control : Subsystem
  "wref, Vref" : Outport
  wires:
  Bus Selector1/1 -> PQ control/2(P (pu)), PV control/2(P (pu))  "<Output active power   Peo (pu)>"
  gen_m/1 -> Bus Selector1/1
  PQ control/1(w_ref (pu)) -> Mux1/1
  PQ control/2(V_ref (pu)) -> Mux1/2
  PV control/1(w_ref (pu)) -> Mux2/1
  set_vtref/1 -> Mux2/2, Mux3/2
  Mux1/1 -> Multiport Switch/2
  Mux2/1 -> Multiport Switch/3
  Mux3/1 -> Multiport Switch/4
  Pref/1 -> PQ control/1(P_ref (pu)), PV control/1(P_ref (pu))
  Bus Selector1/2 -> PQ control/4(Q (pu))  "<Output reactive power  Qeo (pu)>"
  set_wref/1 -> Mux3/1
  Qref/1 -> PQ control/3(Q_ref (pu))
  mode/1 -> Multiport Switch/1
  Multiport Switch/1 -> "wref, Vref"/1

== system HIL_GenSet/GenSet_900kW_07232015/StabilityL ==
  Constant Load : powerlib/Elements/Three-Phase Parallel RLC Load  LConnTagsString=A|B|C  Configuration=Y (grounded)  NominalVoltage=v  NominalFrequency=60  ActivePower=kVA*1E3*pf  InductivePower=kVA*1E3*sqrt(1-pf^2)  CapacitivePower=0  Measurements=None  LoadType=constant Z
  A : PMIOPort  Port=1  Side=Left
  B : PMIOPort  Port=2  Side=Left
  C : PMIOPort  Port=3  Side=Left
  connections:
  A/RConn1 -- Constant Load/LConn1
  B/RConn1 -- Constant Load/LConn2
  C/RConn1 -- Constant Load/LConn3

== system HIL_GenSet/GenSet_900kW_RTLAB/Generator with  Primary Controllers1 ==
  wref : Inport
  Vtref : Inport  Port=2
  Enable : Inport  Port=3
  72.5 kva Diesel Engine Speed & Voltage Control fast : Subsystem
  Synchronous Machine pu Fundamental : powerlib/Machines/Synchronous Machine pu Fundamental  PresetModel=22: 60Hz 460V 1075kVA 1800RPM  MechanicalLoad=Mechanical power Pm  ShowDetailedParameters=on  RotorType=Salient-pole  NominalParameters=[1.075e+006 460 60]  Stator=[0.01524 0.08 2.81 1.64]  Field=[0.004319 0.531]  Dampers2=[0.0652, 0.5134, 0.0287, 0.2553, 7.765e-3, 0.9167 ]  Dampers1=[0.2343 2.655 0.03365 0.2408]  Mechanical=[0.3222 0.01322 2]  PolePairs=2  InitialConditions="[ 0  0  0  0  0  0  0  0  0 ]"  SetSaturation=off  Saturation=[0.6404,0.7127,0.8441,0.9214,0.9956,1.082,1.19,1.316,1.457;0.7,0.7698,0.8872,0.9466,0.9969,1.046,1.1,1.151,1.201]  Units=per unit fundamental parameters  LoadFlowParameters=[1,0,0,0,0]  TsPowergui=0  TsBlock=-1  IterativeModel=Forward Euler  BusType=PV  Pref=0  Qref=0  Qmin=-inf  Qmax=inf  PLF=0  QLF=0
  A : PMIOPort  Port=1  Side=Right
  B : PMIOPort  Port=2  Side=Right
  C : PMIOPort  Port=3  Side=Right
  m : Outport
  wires:
  Enable/1 -> 72.5 kva Diesel Engine Speed & Voltage Control fast/4(Generator Enable)
  Vtref/1 -> 72.5 kva Diesel Engine Speed & Voltage Control fast/2(Vtref)
  wref/1 -> 72.5 kva Diesel Engine Speed & Voltage Control fast/1(wref)
  Synchronous Machine pu Fundamental/1 -> m/1, 72.5 kva Diesel Engine Speed & Voltage Control fast/3(m)
  72.5 kva Diesel Engine Speed & Voltage Control fast/2(Vf) -> Synchronous Machine pu Fundamental/2
  72.5 kva Diesel Engine Speed & Voltage Control fast/1(Pm) -> Synchronous Machine pu Fundamental/1
  connections:
  C/RConn1 -- Synchronous Machine pu Fundamental/RConn3
  B/RConn1 -- Synchronous Machine pu Fundamental/RConn2
  A/RConn1 -- Synchronous Machine pu Fundamental/RConn1

== system HIL_GenSet/GenSet_900kW_RTLAB/PQ control ==
  P_ref (pu) : Inport
  P (pu) : Inport  Port=2
  Q_ref (pu) : Inport  Port=3
  Q (pu) : Inport  Port=4
  Discrete PID Controller : simulink/Continuous/PID Controller  Controller=PID  TimeDomain=Discrete-time  SampleTime=-1  IntegratorMethod=Forward Euler  FilterMethod=Forward Euler  Form=Parallel  P=0.001  I=1  D=0  N=10  InitialConditionSource=internal  InitialConditionForIntegrator=0  InitialConditionForFilter=0  ExternalReset=none  LimitOutput=on  UpperSaturationLimit=1.05  LowerSaturationLimit=0.95  LinearizeAsGain=off  AntiWindupMode=back-calculation  Kb=1  TrackingMode=off  Kt=1  PParamMin=[]  PParamMax=[]  IParamMin=[]  IParamMax=[]  DParamMin=[]  DParamMax=[]  NParamMin=[]  NParamMax=[]  KbParamMin=[]  KbParamMax=[]  KtParamMin=[]  KtParamMax=[]  POutMin=[]  POutMax=[]  IOutMin=[]  IOutMax=[]  DOutMin=[]  DOutMax=[]  NOutMin=[]  NOutMax=[]  KbOutMin=[]  KbOutMax=[]  KtOutMin=[]  KtOutMax=[]  IntegratorOutMin=[]  IntegratorOutMax=[]  FilterOutMin=[]  FilterOutMax=[]  SumOutMin=[]  SumOutMax=[]  SumI1OutMin=[]  SumI1OutMax=[]  SumI2OutMin=[]  SumI2OutMax=[]  SumI3OutMin=[]  SumI3OutMax=[]  SumDOutMin=[]  SumDOutMax=[]  SaturationOutMin=[]  SaturationOutMax=[]  IntegratorContinuousStateAttributes=''  IntegratorStateMustResolveToSignalObject=off  IntegratorRTWStateStorageClass=Auto  FilterContinuousStateAttributes=''  FilterStateMustResolveToSignalObject=off  FilterRTWStateStorageClass=Auto
  Discrete PID Controller1 : simulink/Continuous/PID Controller  Controller=PID  TimeDomain=Discrete-time  SampleTime=-1  IntegratorMethod=Forward Euler  FilterMethod=Forward Euler  Form=Parallel  P=1.2  I=0.5  D=0  N=10  InitialConditionSource=internal  InitialConditionForIntegrator=0  InitialConditionForFilter=0  ExternalReset=none  LimitOutput=on  UpperSaturationLimit=1.05  LowerSaturationLimit=0.95  LinearizeAsGain=off  AntiWindupMode=back-calculation  Kb=1  TrackingMode=off  Kt=1  PParamMin=[]  PParamMax=[]  IParamMin=[]  IParamMax=[]  DParamMin=[]  DParamMax=[]  NParamMin=[]  NParamMax=[]  KbParamMin=[]  KbParamMax=[]  KtParamMin=[]  KtParamMax=[]  POutMin=[]  POutMax=[]  IOutMin=[]  IOutMax=[]  DOutMin=[]  DOutMax=[]  NOutMin=[]  NOutMax=[]  KbOutMin=[]  KbOutMax=[]  KtOutMin=[]  KtOutMax=[]  IntegratorOutMin=[]  IntegratorOutMax=[]  FilterOutMin=[]  FilterOutMax=[]  SumOutMin=[]  SumOutMax=[]  SumI1OutMin=[]  SumI1OutMax=[]  SumI2OutMin=[]  SumI2OutMax=[]  SumI3OutMin=[]  SumI3OutMax=[]  SumDOutMin=[]  SumDOutMax=[]  SaturationOutMin=[]  SaturationOutMax=[]  IntegratorContinuousStateAttributes=''  IntegratorStateMustResolveToSignalObject=off  IntegratorRTWStateStorageClass=Auto  FilterContinuousStateAttributes=''  FilterStateMustResolveToSignalObject=off  FilterRTWStateStorageClass=Auto
  Sum : Sum  Inputs=|-+
  Sum1 : Sum  Inputs=|-+
  w_ref (pu) : Outport
  V_ref (pu) : Outport  Port=2
  wires:
  Q_ref (pu)/1 -> Sum1/2
  Discrete PID Controller1/1 -> V_ref (pu)/1
  Q (pu)/1 -> Sum1/1
  Sum1/1 -> Discrete PID Controller1/1
  P_ref (pu)/1 -> Sum/2
  Discrete PID Controller/1 -> w_ref (pu)/1
  P (pu)/1 -> Sum/1
  Sum/1 -> Discrete PID Controller/1

== system HIL_GenSet/GenSet_900kW_RTLAB/PV control ==
  P_ref (pu) : Inport
  P (pu) : Inport  Port=2
  Discrete PID Controller : simulink/Continuous/PID Controller  Controller=PID  TimeDomain=Discrete-time  SampleTime=-1  IntegratorMethod=Forward Euler  FilterMethod=Forward Euler  Form=Parallel  P=0.001  I=1  D=0  N=10  InitialConditionSource=internal  InitialConditionForIntegrator=0  InitialConditionForFilter=0  ExternalReset=none  LimitOutput=on  UpperSaturationLimit=1.05  LowerSaturationLimit=0.95  LinearizeAsGain=off  AntiWindupMode=back-calculation  Kb=1  TrackingMode=off  Kt=1  PParamMin=[]  PParamMax=[]  IParamMin=[]  IParamMax=[]  DParamMin=[]  DParamMax=[]  NParamMin=[]  NParamMax=[]  KbParamMin=[]  KbParamMax=[]  KtParamMin=[]  KtParamMax=[]  POutMin=[]  POutMax=[]  IOutMin=[]  IOutMax=[]  DOutMin=[]  DOutMax=[]  NOutMin=[]  NOutMax=[]  KbOutMin=[]  KbOutMax=[]  KtOutMin=[]  KtOutMax=[]  IntegratorOutMin=[]  IntegratorOutMax=[]  FilterOutMin=[]  FilterOutMax=[]  SumOutMin=[]  SumOutMax=[]  SumI1OutMin=[]  SumI1OutMax=[]  SumI2OutMin=[]  SumI2OutMax=[]  SumI3OutMin=[]  SumI3OutMax=[]  SumDOutMin=[]  SumDOutMax=[]  SaturationOutMin=[]  SaturationOutMax=[]  IntegratorContinuousStateAttributes=''  IntegratorStateMustResolveToSignalObject=off  IntegratorRTWStateStorageClass=Auto  FilterContinuousStateAttributes=''  FilterStateMustResolveToSignalObject=off  FilterRTWStateStorageClass=Auto
  Sum : Sum  Inputs=|-+
  w_ref (pu) : Outport
  wires:
  Sum/1 -> Discrete PID Controller/1
  P (pu)/1 -> Sum/1
  Discrete PID Controller/1 -> w_ref (pu)/1
  P_ref (pu)/1 -> Sum/2

== system HIL_GenSet/GenSet_900kW_RTLAB2/60kW Generator with  Primary Controllers ==
  note: Mirjana M: Parameters for this generators are preset parameters from SimPower System for 72.5kVAr
  wref : Inport
  Vtref : Inport  Port=2
  Enable : Inport  Port=3
  w_meas_Woodward : Inport  Port=4
  V_meas_Woodward : Inport  Port=5
  72.5 kva Diesel Engine Speed & Voltage Control fast : Subsystem
  Scope2 : Scope  NumInputPorts=2
      settings: YMin=0.949571~0.99979  YMax=1.04953~1  SaveName=ScopeData6
  Synchronous Machine pu Fundamental : powerlib/Machines/Synchronous Machine pu Fundamental  PresetModel=22: 60Hz 460V 1075kVA 1800RPM  MechanicalLoad=Mechanical power Pm  ShowDetailedParameters=on  RotorType=Salient-pole  NominalParameters=[1.075e+006 460 60]  Stator=[0.01524 0.08 2.81 1.64]  Field=[0.004319 0.531]  Dampers2=[0.0652, 0.5134, 0.0287, 0.2553, 7.765e-3, 0.9167 ]  Dampers1=[0.2343 2.655 0.03365 0.2408]  Mechanical=[0.3222 0.01322 2]  PolePairs=2  InitialConditions="[ 0  0  0  0  0  0  0  0  0 ]"  SetSaturation=off  Saturation=[0.6404,0.7127,0.8441,0.9214,0.9956,1.082,1.19,1.316,1.457;0.7,0.7698,0.8872,0.9466,0.9969,1.046,1.1,1.151,1.201]  Units=per unit fundamental parameters  LoadFlowParameters=[1,0,0,0,0]  TsPowergui=0  TsBlock=-1  IterativeModel=Forward Euler  BusType=PV  Pref=0  Qref=0  Qmin=-inf  Qmax=inf  PLF=0  QLF=0
  A : PMIOPort  Port=1  Side=Right
  B : PMIOPort  Port=2  Side=Right
  C : PMIOPort  Port=3  Side=Right
  m : Outport
  wires:
  Enable/1 -> 72.5 kva Diesel Engine Speed & Voltage Control fast/3(Generator Enable)
  Vtref/1 -> 72.5 kva Diesel Engine Speed & Voltage Control fast/2(Vtref)
  wref/1 -> 72.5 kva Diesel Engine Speed & Voltage Control fast/1(wref)
  72.5 kva Diesel Engine Speed & Voltage Control fast/3(Vt) -> Scope2/1
  72.5 kva Diesel Engine Speed & Voltage Control fast/4(w) -> Scope2/2
  Synchronous Machine pu Fundamental/1 -> m/1, 72.5 kva Diesel Engine Speed & Voltage Control fast/4(m)
  72.5 kva Diesel Engine Speed & Voltage Control fast/2(Vf) -> Synchronous Machine pu Fundamental/2
  72.5 kva Diesel Engine Speed & Voltage Control fast/1(Pm) -> Synchronous Machine pu Fundamental/1
  w_meas_Woodward/1 -> 72.5 kva Diesel Engine Speed & Voltage Control fast/5(w_meas_Wood)
  V_meas_Woodward/1 -> 72.5 kva Diesel Engine Speed & Voltage Control fast/6(V_meas_Wood)
  connections:
  C/RConn1 -- Synchronous Machine pu Fundamental/RConn3
  B/RConn1 -- Synchronous Machine pu Fundamental/RConn2
  A/RConn1 -- Synchronous Machine pu Fundamental/RConn1

== system HIL_GenSet/GenSet_900kW_RTLAB2/Interface between Woodward Controller and simated generator ==
  note: Note: This may need a different scaling because it is the reference signal.
      | Reference has to be between 0.95 and 1.05 pu in order to be in tolerance.
  Woodward for wref : Inport
  Woodward for Vref : Inport  Port=2
  Add2 : Sum
  Add3 : Sum
  Gain2 : Gain  Gain=0.005
  Gain3 : Gain  Gain=0.005
  Mux1 : Mux  Inputs=2
  Vref_set : Constant
  wref_set : Constant
  wref,Vref : Outport
  wires:
  Gain2/1 -> Add2/1  "bias"
  Add2/1 -> Mux1/1
  wref_set/1 -> Add2/2
  Gain3/1 -> Add3/1  "bias"
  Vref_set/1 -> Add3/2
  Add3/1 -> Mux1/2
  Woodward for wref/1 -> Gain2/1
  Mux1/1 -> wref,Vref/1  "hardware"
  Woodward for Vref/1 -> Gain3/1

== system HIL_GenSet/GenSet_900kW_RTLAB2/Simulated Generator Controller ==
  Bus Selector1 : BusSelector  OutputSignals="Output active power   Peo (pu),Output reactive power  Qeo (pu)"
  Multiport Switch : MultiPortSwitch  zeroidx=off
  Mux1 : Mux  Inputs=2
  Mux2 : Mux  Inputs=2
  Mux3 : Mux  Inputs=2
  PQ control : Subsystem
  PV control : Subsystem
  Pref : Constant  Value=set_Pref
  Qref : Constant  Value=set_Qref
  mode (1-3) : Constant  Value=mode
  set_vtref : Constant  Value=set_vref
  set_wref : Constant  Value=set_wref
  "wref, Vref" : Outport
  wires:
  Bus Selector1/1 -> PQ control/2(P (pu)), PV control/2(P (pu))  "<Output active power   Peo (pu)>"
  [gen_m] -> Bus Selector1/1
  PQ control/1(w_ref (pu)) -> Mux1/1
  PQ control/2(V_ref (pu)) -> Mux1/2
  PV control/1(w_ref (pu)) -> Mux2/1
  set_vtref/1 -> Mux2/2, Mux3/2
  Mux1/1 -> Multiport Switch/2
  Mux2/1 -> Multiport Switch/3
  Mux3/1 -> Multiport Switch/4
  Pref/1 -> PQ control/1(P_ref (pu)), PV control/1(P_ref (pu))
  Bus Selector1/2 -> PQ control/4(Q (pu))  "<Output reactive power  Qeo (pu)>"
  set_wref/1 -> Mux3/1
  Qref/1 -> PQ control/3(Q_ref (pu))
  mode (1-3)/1 -> Multiport Switch/1
  Multiport Switch/1 -> "wref, Vref"/1

== system HIL_GenSet/GenSet_900kW_nPID_Manual_RTLAB/60kW Generator with  Primary Controllers ==
  note: Mirjana M: Parameters for this generators are preset parameters from SimPower System for 72.5kVAr
  wref : Inport
  Vtref : Inport  Port=2
  Enable : Inport  Port=3
  w_meas_Woodward : Inport  Port=4
  V_meas_Woodward : Inport  Port=5
  72.5 kva Diesel Engine Speed & Voltage Control fast : Subsystem
  Synchronous Machine pu Fundamental : powerlib/Machines/Synchronous Machine pu Fundamental  PresetModel=22: 60Hz 460V 1075kVA 1800RPM  MechanicalLoad=Mechanical power Pm  ShowDetailedParameters=on  RotorType=Salient-pole  NominalParameters=[1.075e+006 460 60]  Stator=[0.01524 0.08 2.81 1.64]  Field=[0.004319 0.531]  Dampers2=[0.0652, 0.5134, 0.0287, 0.2553, 7.765e-3, 0.9167 ]  Dampers1=[0.2343 2.655 0.03365 0.2408]  Mechanical=[0.3222 0.01322 2]  PolePairs=2  InitialConditions="[ 0  0  0  0  0  0  0  0  0 ]"  SetSaturation=off  Saturation=[0.6404,0.7127,0.8441,0.9214,0.9956,1.082,1.19,1.316,1.457;0.7,0.7698,0.8872,0.9466,0.9969,1.046,1.1,1.151,1.201]  Units=per unit fundamental parameters  LoadFlowParameters=[1,0,0,0,0]  TsPowergui=0  TsBlock=-1  IterativeModel=Forward Euler  BusType=PV  Pref=0  Qref=0  Qmin=-inf  Qmax=inf  PLF=0  QLF=0
  Terminator : Terminator
  Terminator1 : Terminator
  A : PMIOPort  Port=1  Side=Right
  B : PMIOPort  Port=2  Side=Right
  C : PMIOPort  Port=3  Side=Right
  m : Outport
  wires:
  Enable/1 -> 72.5 kva Diesel Engine Speed & Voltage Control fast/3(Generator Enable)
  Vtref/1 -> 72.5 kva Diesel Engine Speed & Voltage Control fast/2(Vtref)
  wref/1 -> 72.5 kva Diesel Engine Speed & Voltage Control fast/1(wref)
  72.5 kva Diesel Engine Speed & Voltage Control fast/3(Vt) -> Terminator/1
  72.5 kva Diesel Engine Speed & Voltage Control fast/4(w) -> Terminator1/1
  Synchronous Machine pu Fundamental/1 -> m/1, 72.5 kva Diesel Engine Speed & Voltage Control fast/4(m)
  72.5 kva Diesel Engine Speed & Voltage Control fast/2(Vf) -> Synchronous Machine pu Fundamental/2
  72.5 kva Diesel Engine Speed & Voltage Control fast/1(Pm) -> Synchronous Machine pu Fundamental/1
  w_meas_Woodward/1 -> 72.5 kva Diesel Engine Speed & Voltage Control fast/5(w_meas_Wood)
  V_meas_Woodward/1 -> 72.5 kva Diesel Engine Speed & Voltage Control fast/6(V_meas_Wood)
  connections:
  C/RConn1 -- Synchronous Machine pu Fundamental/RConn3
  B/RConn1 -- Synchronous Machine pu Fundamental/RConn2
  A/RConn1 -- Synchronous Machine pu Fundamental/RConn1
